simulink model "ACC"  (R2022b)
settings: Solver=ode45  StartTime=0.0  StopTime=30  RelTol=1e-3  EnableMultiTasking=on
values from neighbouring files (symbols this model uses):
  alpha_in = 0    [ACCparams.mat]
  C = 1.5    [tut5.m]
  Cd = 0.3    [ACCparams.mat]
  E = 200    [ACCparams.mat]
  Fl = 1000    [ACCparams.mat]    (also in tut5.m = 0)
  G = 4    [ACCparams.mat]    (also in assignment1.m = H + D)
  Ki = 1    [ACCparams.mat]    (also in tut5.m = 1.5)
  Kp = 1    [ACCparams.mat]    (also in tut5.m = 2)
  M = 1500    [ACCparams.mat]
  n = size(A,1)    [assignment1.m]    (also in tut5.m = 0.9)
  R = 0.25    [ACCparams.mat]
  T = 0.5    [tut5.m]
  v_in = 15    [ACCparams.mat]
settings Model: Creator=shashisn  LastModifiedBy=prachit
settings SolverCC: AlgebraicLoopSolver=TrustRegion
settings DataIOCC: LimitDataPoints=on  SaveFormat=Array  SignalLoggingSaveFormat=ModelDataLogs  ReturnWorkspaceOutputs=off
settings OptimizationCC: ExpressionDepthLimit=2147483647  LifeSpan=inf
settings DebuggingCC: UnderspecifiedInitializationDetection=Classic  MergeDetectMultiDrivingBlocksExec=none  FcnCallInpInsideContextMsg=warning  UnconnectedInputMsg=warning  UnconnectedOutputMsg=warning  UnconnectedLineMsg=warning  StateNameClashWarn=warning  SFUnexpectedBacktrackingDiag=warning  SFNoUnconditionalDefaultTransitionDiag=warning  SFExecutionAtInitializationDiag=none  SFMachineParentedDataDiag=warning  ArithmeticOperatorsInVariantConditions=warning
settings HardwareCC: ProdBitPerPointer=32  ProdBitPerSizeT=32  ProdBitPerPtrDiffT=32  ProdLargestAtomicFloat=None  ProdIntDivRoundTo=Undefined  ProdEndianess=Unspecified  ProdWordSize=32  ProdHWDeviceType=32-bit Generic
settings ModelReferenceCC: PropagateSignalLabelsOutOfModel=off
settings SFSimCC: SimUseLocalCustomCode=off  CustomCodeUndefinedFunction=UseInterfaceOnly
settings RTWCC: RTWUseLocalCustomCode=off
settings CodeAppCC: StateflowObjectComments=on
settings GRTTargetCC: TargetLangStandard=C89/C90 (ANSI)  CombineOutputUpdateFcns=off  GRTInterface=on
settings ConfigComp: CovMetricSettings=dw  CovSaveCumulativeToWorkspaceVar=on  CovSaveSingleToWorkspaceVar=on

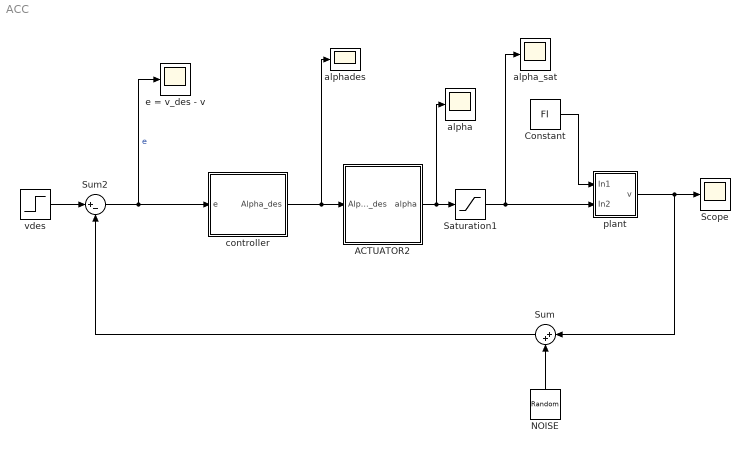
== system ACC ==
  ACTUATOR2 : Subsystem
  Constant : Constant  Value=Fl
  NOISE : RandomNumber  Mean=0.5  Variance=0.01  SampleTime=0.1
  Saturation1 : Saturate  UpperLimit=pi()/2  LowerLimit=-pi()/2
  Scope : Scope
  Sum : Sum  Inputs=|++
  Sum2 : Sum  Inputs=|+-
  alpha : Scope
  alpha_sat : Scope
  alphades : Scope
  controller : Subsystem
  e = v_des - v : Scope
  plant : Subsystem
  vdes : Step  Before=15  After=16  SampleTime=0
  wires:
  Sum2/1 -> controller/1(e), e = v_des - v/1  "e"
  vdes/1 -> Sum2/1
  Constant/1 -> plant/1(In1)
  Saturation1/1 -> alpha_sat/1, plant/2(In2)
  plant/1(v) -> Sum/1, Scope/1
  Sum/1 -> Sum2/2
  NOISE/1 -> Sum/2
  controller/1(Alpha_des) -> ACTUATOR2/1(Alpha_des), alphades/1
  ACTUATOR2/1(alpha) -> alpha/1, Saturation1/1

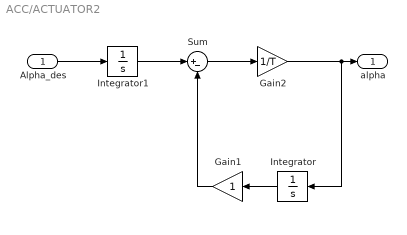
== system ACC/ACTUATOR2 ==
  Alpha_des : Inport
  Gain1 : Gain
  Gain2 : Gain  Gain=1/T
  Integrator : Integrator
  Integrator1 : Integrator
  Sum : Sum  Inputs=|+-
  alpha : Outport
  wires:
  Gain2/1 -> alpha/1, Integrator/1
  Sum/1 -> Gain2/1
  Alpha_des/1 -> Integrator1/1
  Integrator1/1 -> Sum/1
  Integrator/1 -> Gain1/1
  Gain1/1 -> Sum/2

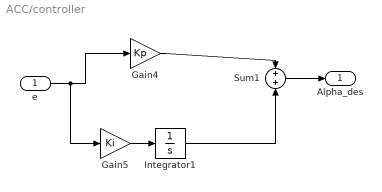
== system ACC/controller ==
  e : Inport
  Gain4 : Gain  Gain=Kp
  Gain5 : Gain  Gain=Ki
  Integrator1 : Integrator  InitialCondition=alpha_in
  Sum1 : Sum  Inputs=+|+
  Alpha_des : Outport
  wires:
  Integrator1/1 -> Sum1/2
  Gain4/1 -> Sum1/1
  Gain5/1 -> Integrator1/1
  e/1 -> Gain5/1, Gain4/1
  Sum1/1 -> Alpha_des/1

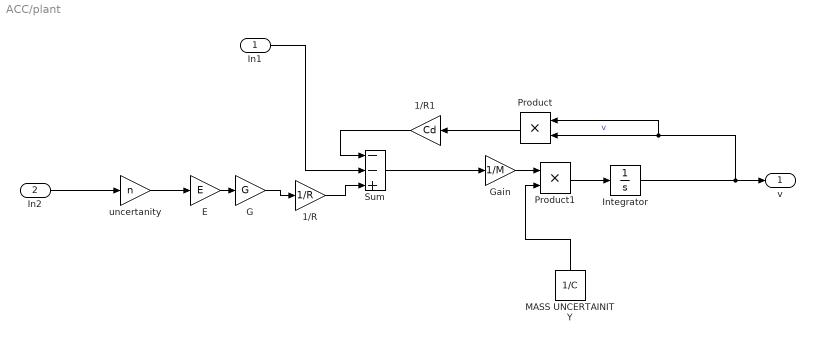
== system ACC/plant ==
  In1 : Inport
  In2 : Inport  Port=2
  1/R : Gain  Gain=1/R
  1/R1 : Gain  Gain=Cd
  E : Gain  Gain=E
  G : Gain  Gain=G
  Gain : Gain  Gain=1/M
  Integrator : Integrator  InitialCondition=v_in
  MASS UNCERTAINITY : Constant  Value=1/C
  Product : Product  RndMeth=Zero
  Product1 : Product
  Sum : Sum  Inputs=--+
  uncertanity : Gain  Gain=n
  v : Outport
  wires:
  G/1 -> 1/R/1
  In1/1 -> Sum/2
  Integrator/1 -> v/1, Product/2, Product/1  "v"
  E/1 -> G/1
  Product/1 -> 1/R1/1
  1/R1/1 -> Sum/1
  1/R/1 -> Sum/3
  In2/1 -> uncertanity/1
  uncertanity/1 -> E/1
  Sum/1 -> Gain/1
  Product1/1 -> Integrator/1
  MASS UNCERTAINITY/1 -> Product1/2
  Gain/1 -> Product1/1
